simulink model "PV_MEV"  (R2025a)
settings: Solver=VariableStepAuto  StartTime=0.0  StopTime=10.0  RelTol=1e-3
InitFcn:
  | init_paras
values from neighbouring files (symbols this model uses):
  C_PFC = 2600e-6    (= 0.0026)    [init_paras.m]
  chg_ctrl_par = [Icc Vcv V_hys T_hys Kp_v_chg Ki_v_chg Kp_i_chg Ki_i_chg Ts_chg D_max_chg t_chg_on k_chg]    [init_paras.m]
  chg_ev = [0 Icc]    [init_paras.m]
  chg_par = [L_chg Voc Rint Ts_chg I_SIGN t_chg_on]    [init_paras.m]
  D = struct('X', {}, 'ti', {}, 'ia', {}, 'tc', {}, 'irms', {}, 'thd', {}, 'trip', {}, 'ttrip', {})    [make_waveform_figs.m]    (also in run_benchmark.m = get_sig('D'))
  det_ema_alpha = 0.1    [init_paras.m]
  det_force = 0    [init_paras.m]
  det_hyst = 0.6    [init_paras.m]
  det_persist = 2    [init_paras.m]
  det_src = 0    [init_paras.m]
  det_t_arm = 0.58    [init_paras.m]
  det_thr = [0.5 0.5 0.5 0.5 0.5]    [init_paras.m]
  det_variant_onehot = double(det_vlist == VARIANT_NAME)    [init_paras.m]
  ENABLE_HIL = 0    [init_paras.m]
  ENABLE_HIL_DET = 0    [init_paras.m]
  ENABLE_HIL_EST = 0    [init_paras.m]
  estimation_src = cfg_row.estimation_src    [init_paras.m]
  Fnom = 50    [init_paras.m]
  Fr_I = Fnom*2    (= 100)    [init_paras.m]
  grid_df = 0    [init_paras.m]
  grid_h5 = 0    [init_paras.m]
  grid_h7 = 0    [init_paras.m]
  grid_var_t0 = 0.7    [init_paras.m]
  hgq_fusion_alpha = [0.6704476522845647 0.7221651725151749 0.6446423751787858 0.41926421682656173]    [init_paras.m]
  hgq_min_ratio = single(0)    [init_paras.m]
  inj_channel = INJ.channel    [init_paras.m]
  inj_dwell = INJ.dwell    [init_paras.m]
  inj_shape = INJ.shape    [init_paras.m]
  inj_t_on = INJ.t_on    [init_paras.m]
  Ki_V = 80    [init_paras.m]
  Kp_I = 0.06    [init_paras.m]
  Kp_V = 0.25    [init_paras.m]
  Kr_I = 2.5    [init_paras.m]
  L_PFC = 600e-6    (= 0.0006)    [init_paras.m]
  Limit_V = 100    [init_paras.m]
  mit_t_ramp = 0.06    [init_paras.m]
  mitigation_mask = 0    [init_paras.m]
  mm_10cycle_points = mm_points_per_cycle * 10    (= 800)    [init_paras.m]
  mm_fund_freq = 50    [init_paras.m]
  mm_points_per_cycle = 80    [init_paras.m]
  R_bleed = 100e3    (= 100000)    [init_paras.m]
  R_pre = Ro*2    (= 44.44)    [init_paras.m]
  res_par = double(RES.par(:)'); end    [init_paras.m]
  RL_PFC = 20e-3    (= 0.02)    [init_paras.m]
  Ro = 22.22    [init_paras.m]
  t_pre_off = 0.30    (= 0.3)    [init_paras.m]
  Ts_chg = 10e-6    (= 1e-05)    [init_paras.m]
  Ts_Control = 1/Fc    [init_paras.m]
  Ts_Power = 50e-9    (= 5e-08)    [init_paras.m]    (also in run_benchmark.m = evalin('base','Ts_Power'))
  use_d_predict = cfg_row.use_d_predict    [init_paras.m]
  use_detector = 0    [init_paras.m]
  use_harmonic = cfg_row.use_harmonic    [init_paras.m]
  use_p_predict = cfg_row.use_p_predict    [init_paras.m]
  Vnom_ac = 240    [init_paras.m]
  vref_ev = [0 0]    [init_paras.m]
undefined symbols (not defined in the file or in its folder): D1, Delta, DiscIntNeverNeededParam
libraries: spsSeriesRLCBranchLib x17, spsMeanLib x16, MyLibrary x12, spsCurrentMeasurementLib x9, spsFourierLib x8, spsTHDLib x8, spsVoltageMeasurementLib x8, spsDiodeLib x7, simulink x7, pycoexlib x5, instrumentlib x4, spsPWMGeneratorDCDCLib x4
(part 7 of 7)

== matlab function PV_MEV/EV System/PFC Control/D_predict ==
  data: i_L input; D output; i_ref input; V_in input; Ts input; L_in input; V_o input; theta_pll input; amp_est input; phase_est input; use_harmonic input
function D  = fcn(i_L, i_ref, V_in, Ts, L_in, V_o, theta_pll, amp_est, phase_est, use_harmonic)

    persistent theta_prev;
    if isempty(theta_prev)
        theta_prev = theta_pll;
    end

    % hyper parameters
    track_gain = 0.35;
    damp_gain = 0.015;

    % Optional
    lead_steps = 1.0;


    % Initialisation 
    L = max(L_in, 1e-9);
    Ts_eff = max(Ts, 1e-9);
    Vo = max(abs(V_o), 1.0);
    ui_L = max(abs(i_L), 1e-6);

    if V_in > 0
        line_sign = 1.0;
    else
        line_sign = -1.0;
    end

    % Keep the sign of i_ref: a negative reference from the voltage loop must reduce
    % the current (D -> 0, same as the PR controller), not demand |i_ref|.
    i_ref_signed = line_sign * i_ref;

    plant_gain = line_sign * L / (Vo * Ts_eff);
    D_ff = 1.0 - abs(V_in) / Vo;

    if use_harmonic

        dtheta = atan2(sin(theta_pll - theta_prev), cos(theta_pll - theta_prev));
        theta_prev = theta_pll;

        omega_inst = dtheta / Ts_eff;

        theta_ctrl = theta_pll + omega_inst * Ts_eff * lead_steps;

        A3 = abs(amp_est(2));
        A5 = abs(amp_est(3));
        A7 = abs(amp_est(4));

        phi3 = phase_est(1);
        phi5 = phase_est(2);
        phi7 = phase_est(3);

        phase_sign = 1.0;

        ih3 = A3 * sin(3.0 * theta_ctrl + phase_sign * phi3);
        ih5 = A5 * sin(5.0 * theta_ctrl + phase_sign * phi5);
        ih7 = A7 * sin(7.0 * theta_ctrl + phase_sign * phi7);

        k3 = 1.00;
        k5 = 1.08;
        k7 = 1.00;

        ih_357 = k3 * ih3 + k5 * ih5 + k7 * ih7;

        i_ref_signed = i_ref_signed - ih_357;
    end

    i_err = i_ref_signed - i_L;

    D_corr = plant_gain * track_gain * i_err;
    D_damp = -line_sign * damp_gain * (i_L - i_ref_signed) / ui_L;

    D = D_ff + D_corr + D_damp;
end

== matlab function PV_MEV/EV System2/PFC Control/fft estimation 1 cycle2/FFT_estimation_1 ==
  data: u input; amp output; phase output; fs input; f0 input
function [amp, phase] = FFT_estimation_1(u, fs, f0)
%#codegen

x = double(u(:));
N = length(x);

h = zeros(4, 1);
h(1) = 1;
h(2) = 3;
h(3) = 5;
h(4) = 7;

X = fft(x);

amp = zeros(4, 1);
phase_abs_sin = zeros(4, 1);
phase = zeros(3, 1);

tol = 1e-12;

for i = 1:4
    harmonicOrder = h(i);

    bin = round(harmonicOrder * f0 * double(N) / fs);

    if bin <= 0 || bin > floor(double(N) / 2)
        amp(i) = 0;
        phase_abs_sin(i) = 0;
    else
        idx = int32(bin + 1);
        C = X(idx);

        if mod(N, 2) == 0 && bin == N / 2
            amp(i) = abs(C) / double(N);
        else
            amp(i) = 2 * abs(C) / double(N);
        end

        if amp(i) < tol
            phase_abs_sin(i) = 0;
        else
            ph_raw = angle(C);

            ph_sin = ph_raw + pi/2;

            phase_abs_sin(i) = atan2(sin(ph_sin), cos(ph_sin));
        end
    end
end

if amp(1) < tol
    phase(1) = 0;
    phase(2) = 0;
    phase(3) = 0;
else
    phase(1) = atan2( ...
        sin(phase_abs_sin(2) - 3 * phase_abs_sin(1)), ...
        cos(phase_abs_sin(2) - 3 * phase_abs_sin(1)) ...
    );

    phase(2) = atan2( ...
        sin(phase_abs_sin(3) - 5 * phase_abs_sin(1)), ...
        cos(phase_abs_sin(3) - 5 * phase_abs_sin(1)) ...
    );

    phase(3) = atan2( ...
        sin(phase_abs_sin(4) - 7 * phase_abs_sin(1)), ...
        cos(phase_abs_sin(4) - 7 * phase_abs_sin(1)) ...
    );
end

end

== matlab function PV_MEV/EV System2/PFC Control/fft estimation 10 cycle2/FFT_estimation ==
  data: u input; amp output; phase output; fs input; f0 input
function [amp, phase] = FFT_estimation(u, fs, f0)
%#codegen

x = double(u(:));
N = length(x);

h = zeros(4, 1);
h(1) = 1;
h(2) = 3;
h(3) = 5;
h(4) = 7;

X = fft(x);

amp = zeros(4, 1);
phase_abs_sin = zeros(4, 1);
phase = zeros(3, 1);

tol = 1e-12;

for i = 1:4
    harmonicOrder = h(i);

    bin = round(harmonicOrder * f0 * double(N) / fs);

    if bin <= 0 || bin > floor(double(N) / 2)
        amp(i) = 0;
        phase_abs_sin(i) = 0;
    else
        idx = int32(bin + 1);
        C = X(idx);

        if mod(N, 2) == 0 && bin == N / 2
            amp(i) = abs(C) / double(N);
        else
            amp(i) = 2 * abs(C) / double(N);
        end

        if amp(i) < tol
            phase_abs_sin(i) = 0;
        else
            ph_raw = angle(C);

            ph_sin = ph_raw + pi/2;

            phase_abs_sin(i) = atan2(sin(ph_sin), cos(ph_sin));
        end
    end
end

if amp(1) < tol
    phase(1) = 0;
    phase(2) = 0;
    phase(3) = 0;
else
    phase(1) = atan2( ...
        sin(phase_abs_sin(2) - 3 * phase_abs_sin(1)), ...
        cos(phase_abs_sin(2) - 3 * phase_abs_sin(1)) ...
    );

    phase(2) = atan2( ...
        sin(phase_abs_sin(3) - 5 * phase_abs_sin(1)), ...
        cos(phase_abs_sin(3) - 5 * phase_abs_sin(1)) ...
    );

    phase(3) = atan2( ...
        sin(phase_abs_sin(4) - 7 * phase_abs_sin(1)), ...
        cos(phase_abs_sin(4) - 7 * phase_abs_sin(1)) ...
    );
end

end

== matlab function PV_MEV/EV System/PFC Control/HGQ FFT-DL Hybrid ==
  data: fft_amplitude input size=[4 1]; amplitude_out output size=[4 1]; fft_phase input size=[3 1]; dl_amplitude input size=[4 1]; dl_phase input size=[3 1]; alpha input size=[4 1]; minimum_ratio input size=1; phase_out output size=[3 1]; dl_accepted output size=1
function [amplitude_out, phase_out, dl_accepted] = harmonic_hybrid_fusion_block(fft_amplitude, fft_phase, dl_amplitude, dl_phase, alpha, minimum_ratio)
%#codegen
% Fuse FFT (1-cycle) and HGQ2 harmonic estimates in Cartesian coordinates with a
% per-order weight alpha; falls back to FFT when the DL output fails the watchdog.
amplitude_out = zeros(4, 1, 'single');
phase_out = zeros(3, 1, 'single');
dl_accepted = false;
fft_amp = zeros(4, 1, 'single'); dl_amp = zeros(4, 1, 'single'); weight = zeros(4, 1, 'single');
fft_phi = zeros(3, 1, 'single'); dl_phi = zeros(3, 1, 'single');
for index = 1:4
    fft_amp(index) = single(fft_amplitude(index)); dl_amp(index) = single(dl_amplitude(index));
    weight(index) = min(max(single(alpha(index)), single(0)), single(1));
end
for index = 1:3
    fft_phi(index) = single(fft_phase(index)); dl_phi(index) = single(dl_phase(index));
end
ratio = max(single(minimum_ratio), single(0));
valid = true;
for index = 1:4
    valid = valid && isfinite(dl_amp(index)) && dl_amp(index) >= single(0);
end
for index = 1:3
    valid = valid && isfinite(dl_phi(index));
end
valid = valid && dl_amp(1) > single(1e-5);
valid = valid && max(dl_amp(2:4)) <= single(4) * max(dl_amp(1), single(1e-5));
if ~valid
    amplitude_out = fft_amp; phase_out = fft_phi;
    return
end
dl_accepted = true;
amplitude_out(1) = (single(1) - weight(1)) * fft_amp(1) + weight(1) * dl_amp(1);
for index = 1:3
    harmonic = index + 1;
    real_part = (single(1) - weight(harmonic)) * fft_amp(harmonic) * cos(fft_phi(index)) + weight(harmonic) * dl_amp(harmonic) * cos(dl_phi(index));
    imag_part = (single(1) - weight(harmonic)) * fft_amp(harmonic) * sin(fft_phi(index)) + weight(harmonic) * dl_amp(harmonic) * sin(dl_phi(index));
    amplitude_out(harmonic) = hypot(real_part, imag_part);
    phase_out(index) = atan2(imag_part, real_part);
    if amplitude_out(harmonic) < ratio * max(amplitude_out(1), single(1e-5))
        amplitude_out(harmonic) = single(0); phase_out(index) = fft_phi(index);
    end
end
end

== matlab function PV_MEV/EV System/PFC Control/EMI Detector/emi_features ==
  data: X input size=[200 12]; f output size=[1 48]
function f = emi_features(X)
%#codegen
persistent prev
if isempty(prev), prev = zeros(1, 36); end
n = size(X, 1);
vdc = X(:,1); vac = X(:,2); iac = X(:,3); iref = X(:,4); th = X(:,5); d = X(:,6); vr = X(:,7);
vbat = X(:,8); ibat = X(:,9); ddc = X(:,10); st = X(:,11); irb = X(:,12);
k = (0:n-1)';
w1 = 2*pi/n; c1 = cos(w1*k); s1 = sin(w1*k); c2 = cos(2*w1*k); s2 = sin(2*w1*k); c3 = cos(3*w1*k); s3 = sin(3*w1*k);
vac_amp = 2/n*hypot(vac'*c1, vac'*s1); vac_mean = mean(vac);
h1 = 2/n*hypot(iac'*c1, iac'*s1); h2 = 2/n*hypot(iac'*c2, iac'*s2); h3 = 2/n*hypot(iac'*c3, iac'*s3);
iac_mean = mean(iac); iac_rms = sqrt(mean(iac.^2)); pos = max(iac); neg = min(iac);
ref = iref .* abs(sin(th)) .* sign(sin(th));
if std(ref) > 1e-6 && std(iac) > 1e-6, cc = sum((iac-mean(iac)).*(ref-mean(ref))) / (n*std(iac,1)*std(ref,1)); else, cc = 0; end
ref_err = sqrt(mean((abs(iac) - abs(ref)).^2)) / max(iac_rms, 1e-3);
ph_i = atan2(-(iac'*s1), iac'*c1); ph_v = atan2(-(vac'*s1), vac'*c1); dphi = angle(exp(1i*(ph_i - ph_v)));
vdc_mean = mean(vdc); vdc_rip = max(vdc) - min(vdc); vdc_err = vdc_mean - mean(vr);
d_ff = 1 - abs(vac) ./ max(vdc, 50);
p_ac = mean(vac.*iac); p_chg = mean(vbat.*ibat); p_ratio = p_chg / max(p_ac, 50);
vbm = mean(vbat); ddm = mean(ddc);
row = [vac_mean, vac_amp, vac_mean/max(vac_amp,1), iac_mean, iac_rms, pos, neg, pos+neg, h2/max(h1,1e-3), h3/max(h1,1e-3), h1, ...
       cc, ref_err, iac_mean/max(h1,1e-3), dphi, vdc_mean, vdc_rip, vdc_err, mean(iref), min(iref), max(iref), mean(iref < 0), mean(d), mean(d) - mean(d_ff), ...
       vbm, mean(ibat), ddm, mean(st), mean(irb), max(vbat)-min(vbat), max(ibat)-min(ibat), p_ac, p_chg, p_ratio, ...
       ddm*vdc_mean/max(vbm,50) - 1, vbm - ddm*vdc_mean];
if all(prev == 0)
    dl = zeros(1, 7);
else
    dl = [row(16)-prev(16), row(19)-prev(19), row(5)-prev(5), row(4)-prev(4), row(25)-prev(25), row(26)-prev(26), row(34)-prev(34)];
end
prev = row;
% v3 extras (features.FEATURE_NAMES_V3_EXTRA): bus 50 Hz ripple, its ratio to the 100 Hz ripple, its phase vs Vac, duty half-cycle asymmetry, pad
vh1 = 2/n*hypot(vdc'*c1, vdc'*s1); vh2 = 2/n*hypot(vdc'*c2, vdc'*s2);
vph = angle(exp(1i*(atan2(-(vdc'*s1), vdc'*c1) - ph_v)));
sp = sin(th) > 0; sn = sin(th) < 0; dp = 0; dn = 0; if any(sp), dp = mean(d(sp)); end; if any(sn), dn = mean(d(sn)); end
f = [row, dl, vh1, vh1/max(vh2, 0.1), vph, dp - dn, 0];

== matlab function PV_MEV/EV System/PFC Control/EMI Detector/emi_augment ==
  data: f input size=[1 48]; x output size=[1 48]; st input size=[1 49]; onehot input size=[1 6]; alpha input size=1; stn output size=[1 49]
function [x, stn] = emi_augment(f, st, onehot, alpha)
%#codegen
% st = [ema(1:48), n_cycles_seen]
ema = st(1:48); cnt = st(49);
warm = 3;
if cnt < warm
    ema = (ema*cnt + f) / (cnt + 1);      % running mean of the warm-up cycles
    dev = zeros(1, 48);
else
    dev = f - ema;
    ema = (1 - alpha)*ema + alpha*f;
end
stn = [ema, cnt + 1];
x = f;   % 48 base features only (baseline-relative block and one-hot did not help); dev / onehot kept for later

== matlab function PV_MEV/EV System/PFC Control/EMI Detector/emi_decide ==
  data: raw input size=[1 20]; chan output size=[1 5]; thr input size=[1 5]; persist input size=1; cnt input size=[1 5]; hyst input size=1; flag input size=[1 5]; cls output size=1; conf output size=1; amp output size=[1 5]; cntn output size=[1 5]; flagn output size=[1 5]
function [chan, cls, conf, amp, cntn, flagn] = emi_decide(raw, thr, persist, cnt, hyst, flag)
%#codegen
% raw = [5 channel logits, 10 class logits (unused, zeros), 5 signed normalized amplitudes]
% set a channel after `persist` consecutive cycles >= thr, clear it when p < hyst*thr (hysteresis)
pc = 1 ./ (1 + exp(-double(raw(1:5))));
hit = double(pc >= thr); low = double(pc < hyst .* thr);
cntn = (cnt + 1) .* hit;                 % consecutive cycles above threshold
flagn = flag .* (1 - low) + (1 - flag) .* double(cntn >= persist);
chan = flagn;
z = double(raw(6:15)); z = z - max(z); p = exp(z) / sum(exp(z));
[conf, i] = max(p); cls = i - 1;         % 0 none .. 9 multi (features.CLASSES order)
amp = double(raw(16:20)) .* chan;        % per-channel amplitude (Vdc/100 V, Vac/40 V, Iac/20 A, Vbat/25 V, Ibat/8 A), 0 while not flagged

== matlab function PV_MEV/EV System/PFC Control/Mitigation ==
  data: flags input size=[1 5]; Vdc_fb output size=1; amps input size=[1 5]; Vdc input size=1; Vac input size=1; th input size=1; iL input size=1; Iref input size=1; chg input size=[1 9]; mask input size=1; use_det input size=1; force input size=1; Ts input size=1; t_ramp input size=1; Iref_out output size=1; Vin_out output size=1; iL_out output size=1; hold output size=1; g_alpha output size=1; dbg output size=[1 7]; tnow input size=1; t_arm input size=1; inj_ch input size=[1 3]; inj_sh input size=[1 3]; inj_t0 input size=1; inj_dw input size=1; Ilim0 input double size=1; Ilim output double size=1; Vo_ctl output double size=1
function [Vdc_fb, Iref_out, Vin_out, iL_out, hold, g_alpha, dbg, Ilim, Vo_ctl] = mitigation(flags, amps, Vdc, Vac, th, iL, Iref, chg, mask, use_det, force, Ts, t_ramp, tnow, t_arm, inj_ch, inj_sh, inj_t0, inj_dw, Ilim0)
%#codegen
% Detection-conditioned signal corrections for MPCC_R (build_mitigation.m, build_supp.m).  Runs at Ts_Control.
% flags/amps: detector channel flags and signed normalized amplitudes (Vdc Vac Iac Vbat Ibat)
% chg = [Vbat_real Ibat_real Vbat_int Ibat_int D_dcdc state Iref_bat P_charge Idc]
% force = 1: every flag on (MPCC_R_ON); force = 2: oracle flags from the injection definition (MPCC_R_OR)
% M9 (512): slew-limited introduction / removal of the Vdc correction (bumpless), MPCC_R_B
% M11 (2048): protection-consistent voltage-loop limit Ilim = 55 A (OC 65 A less ripple and an uncorrected DC offset) while any correction is active
% M13 (8192): entry-only slew (1000 V/s) of the bus correction during the first 0.1 s after the Vdc flag rises (M9 acts on the fallback path only)
persistent g dVf Iref_prev pkp pkn Vamp th_prev init eb t_rise
if isempty(init), g = zeros(1, 5); dVf = 0; Iref_prev = 0; pkp = 0; pkn = 0; Vamp = 0; th_prev = 0; eb = 0; t_rise = -1; init = 1; end
M = @(k) bitand(uint32(mask), uint32(2^k)) > 0;
f = flags .* (use_det > 0);
if force == 1, f = ones(1, 5); end
if force > 1
    f = zeros(1, 5); dly = 0.02 * round((force - 2) * 10);   % force = 2.d: oracle flags delayed by d grid cycles (fixed-delay oracle)
    if tnow >= inj_t0 + dly && tnow < inj_t0 + inj_dw + dly
        for i = 1:3, c = inj_ch(i); if c >= 1 && c <= 5 && inj_sh(i) ~= 7, f(c) = 1; end, end
    end
end
if tnow < t_arm, f = zeros(1, 5); end          % detector armed only after start-up (det_t_arm)
if f(1) > 0.5, f(4) = 0; f(5) = 0; end         % priority: a Vdc-chain flag explains the charger-side symptoms (Vbat / Ibat flags are consequences)
% --- channel gains: Vdc immediate (a measurement correction must track the bias, not ramp), the rest ramp out over t_ramp (M7)
g1_prev = g(1);
for c = 1:5
    if f(c) > 0.5, g(c) = 1;
    elseif M(7) && c ~= 1, g(c) = max(0, g(c) - Ts / max(t_ramp, Ts));
    else, g(c) = 0; end
end
if g(1) > 0 && g1_prev == 0, t_rise = tnow; end   % rising edge of the bus correction (M13 entry window)
% --- Vdc chain: bias estimate dV = Vdc_int - Vdc_true
Vbat_i = chg(3); Ibat_i = chg(4); Ddc = chg(5);
dV_det = amps(1) * 100;
phys_ok = (Ddc > 0.3) && (Ddc < 0.98) && (Ibat_i > 1);
if phys_ok
    dV = Vdc - Vbat_i / Ddc;                    % charger duty tells the true bus: Vbat = D_dcdc * Vdc_true
else
    dV = dV_det;
end
dV = min(max(dV, -120), 120);
% --- M10 (1024): baseline-referenced estimate.  The residual seen while no bus flag is up is a model-mismatch offset
% (charger losses, parameter error), not a bias: track it slowly (0.2 s) while it moves by less than 5 V, freeze it
% while a flag is up or the residual jumps (an attack), and remove it from the estimate.
if M(10)
    if tnow < t_arm && phys_ok, eb = eb + (Ts / 0.1) * (dV - eb);                                   % calibration before arming
    elseif g(1) == 0 && phys_ok && abs(dV - eb) < 5, eb = eb + (Ts / 0.2) * (dV - eb); end        % slow tracking, jumps excluded
    if phys_ok, dV = min(max(dV - eb, -120), 120); end
end
Vdc_fb = Vdc;
if M(9) && ~phys_ok
    % bumpless: only the amplitude-head fallback is slew-limited (500 V/s); the physics estimate tracks the true bias and
    % vanishes with it, a rate limit there only delays the correction (E-DC-01b: 50 ms of stale correction -> OV)
    tgt = 0; if g(1) > 0, tgt = dV; end
    lim = 500 * Ts; stp = tgt - dVf; stp = min(max(stp, -lim), lim); dVf = dVf + stp;
    if M(0), Vdc_fb = Vdc - dVf; end
else
    if g(1) > 0
        if M(13) && tnow < t_rise + 0.1
            lim = 1000 * Ts; stp = min(max(dV - dVf, -lim), lim); dVf = dVf + stp;   % M13: the correction enters at 1000 V/s, leaves at once
        else, dVf = dVf + (Ts / 0.005) * (dV - dVf); end
    else, dVf = 0; end
    if M(0), Vdc_fb = Vdc - g(1) * dVf; end
end
% --- M11: while a correction is active the voltage loop may not command a current the protection would trip on
Ilim = Ilim0;
if M(11) && (g(1) > 0 || g(4) > 0), Ilim = 55; end   % only the power-moving corrections M0 / M5 (an Ibat / Iac / Vac flag alone leaves the limit at Limit_V)
% --- M14 (16384): the corrected bus sample also feeds the current predictor (its plant model uses V_o); without it a bus bias
% makes the inner loop deliver a current that differs from the reference and the outer loop must over-command (E-DC-02b)
Vo_ctl = Vdc;
if M(14), Vo_ctl = Vdc_fb; end
% --- Iref amplitude limits (M0 floor, M1 slew) live in the separate block 'Mitigation Iref' (algebraic loop)
Iref_out = 0 * Iref + Iref_prev * 0;
% --- Vac chain: PLL-reconstructed feed-forward voltage (peak-to-peak / 2 of the previous cycle)
if th < th_prev - 3                          % wrap: new cycle
    Vamp = 0.5 * (pkp - pkn); pkp = 0; pkn = 0;
end
th_prev = th; pkp = max(pkp, Vac); pkn = min(pkn, Vac);
Vin_out = Vac;
if M(2) && g(2) > 0 && Vamp > 50, Vin_out = Vac + g(2) * (Vamp * sin(th) - Vac); end
% --- Iac chain: DC compensation of the predictor current, estimator hold
iL_out = iL;
if M(3), iL_out = iL - g(3) * amps(3) * 20; end
hold = 0;
if M(4) && g(3) > 0, hold = 1; end
% --- fusion weight towards the HGQ2 estimate while Vac is flagged
g_alpha = 0;
if M(8), g_alpha = g(2); end
dbg = [g(1), dVf, double(phys_ok), Vamp, g(3), eb, Ilim];

== matlab function PV_MEV/EV System/Charger Stage/batt ==
  data: Ibat input double size=1; Vbat output double size=1; pp input double size=[1 6]; P output double size=1
function [Vbat, P] = batt(Ibat, pp)
% Battery terminal voltage and charging power from the current state.
Vbat = pp(2) + pp(3)*Ibat;
P = Vbat*Ibat;

== matlab function PV_MEV/EV System/Charger Stage/ctrl ==
  data: Vbat_m input double size=1; D output double size=1; Ibat_m input double size=1; Vdc input double size=1; t input double size=1; x input double size=[1 5]; pc input double size=[1 13]; ev input double size=[1 2]; Iref output double size=1; xn output double size=[1 5]; state output double size=1
function [D, Iref, xn, state] = ctrl(Vbat_m, Ibat_m, Vdc, t, x, pc, ev)
% CC/CV charge controller.  x = [state tmr xv xi]  (0 CC, 1 CV)
% pc = [Icc Vcv Vhys Thys Kp_v Ki_v Kp_i Ki_i Ts Dmax t_on k_ramp k_soft]; k_soft > 0 (M12): rising slew limit on Iref at every re-engagement
% ev = [t_step Icc_new]: benign charging-current reference step (t_step <= 0: none)
Icc=pc(1); Vcv=pc(2); Vhys=pc(3); Thys=pc(4); Kpv=pc(5); Kiv=pc(6);
Kpi=pc(7); Kii=pc(8); Ts=pc(9); Dmax=pc(10); t_on=pc(11); kr=pc(12); kso=0; if numel(pc) >= 13, kso=pc(13); end
if ev(1) > 0 && t >= ev(1), Icc = ev(2); end
st = x(1); tmr = x(2); xv = x(3); xi = x(4); Iprev = x(5);
Iramp = min(Icc, max(0, (t - t_on)*kr));
% --- state machine
if st == 0
    if Vbat_m >= Vcv, st = 1; tmr = 0; end
else
    if Vbat_m <= Vcv - Vhys, tmr = tmr + Ts; else, tmr = 0; end
    if tmr >= Thys, st = 0; tmr = 0; end
end
% --- outer voltage loop (CV only), preloaded to Iramp in CC
if st == 1
    ev = Vcv - Vbat_m;
    xv = xv + Kiv*ev*Ts;
    Iref = Kpv*ev + xv;
    if Iref > Iramp, Iref = Iramp; xv = min(xv, Iramp); end
    if Iref < 0,     Iref = 0;     xv = max(xv, 0); end
else
    Iref = Iramp; xv = Iramp;
end
if kso > 0 && t >= t_on && Iref > Iprev + kso*Ts, Iref = Iprev + kso*Ts; xv = min(xv, Iref); end   % M12: soft re-engagement
% --- inner current loop with duty feed-forward
ei = Iref - Ibat_m;
xi = xi + Kii*ei*Ts;
Dff = Vbat_m / max(Vdc, 50);
D = Dff + Kpi*ei + xi;
if D > Dmax, D = Dmax; xi = xi - Kii*ei*Ts; end
if D < 0,    D = 0;    xi = xi - Kii*ei*Ts; end
if t < t_on, D = 0; xi = 0; end
xn = [st tmr xv xi Iref];
state = st;

== matlab function PV_MEV/EV System/Charger Stage/plant ==
  data: D input double size=1; Ibat_next output double size=1; Ibat input double size=1; Vdc input double size=1; pp input double size=[1 6]; t input double size=1; Isrc output double size=1; chg_eff parameter double
function [Ibat_next, Isrc] = plant(D, Ibat, Vdc, pp, t, chg_eff)
% Averaged buck.  pp = [L_chg Voc Rint Ts_chg I_SIGN t_chg_on]
% Ibat is the inductor/battery current state (>= 0, diode conduction).
L = pp(1); Voc = pp(2); Rint = pp(3); Ts = pp(4); sgn = pp(5);
Vbat = Voc + Rint*Ibat;
Idc = D*Ibat;                      % lossless averaged input current
Isrc = sgn*Idc;
if t < pp(6)
    Ibat_next = 0;
else
    Ibat_next = Ibat + Ts/L*(chg_eff*D*Vdc - Vbat);   % chg_eff: conversion loss (model-mismatch test)
    if Ibat_next < 0, Ibat_next = 0; end
end

== matlab function PV_MEV/EV System/Charger Stage/chg_corr ==
  data: Vbat_m input size=1; Vbat_c output size=1; Ibat_m input size=1; flags input size=[1 5]; amps input size=[1 5]; mask input size=1; use_det input size=1; force input size=1; Ts input size=1; t_ramp input size=1; Ibat_c output size=1; tnow input size=1; t_arm input size=1; Vdc input size=1; D_prev input size=1; inj_ch input size=[1 3]; inj_sh input size=[1 3]; inj_t0 input size=1; inj_dw input size=1
function [Vbat_c, Ibat_c] = chg_corr(Vbat_m, Ibat_m, flags, amps, mask, use_det, force, Ts, t_ramp, tnow, t_arm, Vdc, D_prev, inj_ch, inj_sh, inj_t0, inj_dw)
%#codegen
% M5 / M6: remove the detected Vbat / Ibat measurement bias before the CC/CV controller (build_mitigation.m, build_supp.m)
% force = 2: oracle flags from the injection definition; M9 (512): slew-limited (200 V/s) Vbat correction
persistent g dVf init eb
if isempty(init), g = zeros(1, 2); dVf = 0; eb = 0; init = 1; end
fl = flags .* (use_det > 0);
if force == 1, fl = ones(1, 5); end
if force > 1
    fl = zeros(1, 5); dly = 0.02 * round((force - 2) * 10);
    if tnow >= inj_t0 + dly && tnow < inj_t0 + inj_dw + dly
        for i = 1:3, c = inj_ch(i); if c >= 1 && c <= 5 && inj_sh(i) ~= 7, fl(c) = 1; end, end
    end
end
f = fl(4:5);
if tnow < t_arm || fl(1) > 0.5, f = zeros(1, 2); end   % armed after start-up; a Vdc-chain flag overrides the charger-side flags
ramp = bitand(uint32(mask), uint32(128)) > 0;
for c = 1:2
    if f(c) > 0.5, g(c) = 1;
    elseif ramp, g(c) = max(0, g(c) - Ts / max(t_ramp, Ts));
    else, g(c) = 0; end
end
Vbat_c = Vbat_m; Ibat_c = Ibat_m;
phys_ok = (D_prev > 0.3) && (D_prev < 0.98) && (Ibat_m > 1) && (Vdc > 250);
if phys_ok, dV = Vbat_m - D_prev * Vdc; else, dV = amps(4) * 25; end   % buck: Vbat = D * Vdc while regulating; detector amplitude as fallback
dV = min(max(dV, -60), 60);
if bitand(uint32(mask), uint32(1024)) > 0      % M10: baseline-referenced (model-mismatch offset removed), see Mitigation
    if tnow < t_arm && phys_ok, eb = eb + (Ts / 0.1) * (dV - eb);
    elseif g(1) == 0 && phys_ok && abs(dV - eb) < 3, eb = eb + (Ts / 0.2) * (dV - eb); end
    if phys_ok, dV = min(max(dV - eb, -60), 60); end
end
if bitand(uint32(mask), uint32(512)) > 0 && ~phys_ok      % M9: slew-limited amplitude-head fallback only (100 V/s)
    tgt = 0; if g(1) > 0, tgt = dV; end
    lim = 100 * Ts; stp = tgt - dVf; stp = min(max(stp, -lim), lim); dVf = dVf + stp;
    if bitand(uint32(mask), uint32(32)) > 0, Vbat_c = Vbat_m - dVf; end
else
    if g(1) > 0, dVf = dVf + (Ts / 0.002) * (dV - dVf); else, dVf = 0; end
    if bitand(uint32(mask), uint32(32)) > 0, Vbat_c = Vbat_m - g(1) * dVf; end
end
if bitand(uint32(mask), uint32(64)) > 0, Ibat_c = Ibat_m - g(2) * amps(5) * 8; end

== matlab function PV_MEV/EV System/PFC Control/UMPC Function Full bridge1 ==
  data: i_L input; y output; i_ref input; V_in input; Ts input; L_in input; V_o input; g_on output; g_off output
function [y,g_on,g_off]= fcn(i_L, i_ref, V_in, Ts, L_in, V_o)

    L=L_in;

    if V_in >= 0
        i_ref_signed = i_ref;
    else
        i_ref_signed = -i_ref;
    end;

    % -- Positive half Cycle
    if V_in >0
        % --- Candidate 1: Switch ON ---
        g_on  = i_L + (V_in)*Ts/L;
        e_on  = abs(g_on - i_ref_signed);
        
        % --- Candidate 2: Switch OFF ---
        g_off = i_L + (V_in - V_o)*Ts/L;
        e_off = abs(g_off - i_ref_signed);

     % -- Negative half Cycle
    else
        % --- Candidate 1: Switch ON ---
        g_on  = i_L + (V_in)*Ts/L;
        e_on  = abs(g_on - i_ref_signed);

        % --- Candidate 2: Switch OFF ---
        g_off = i_L + (V_in + V_o)*Ts/L;
        e_off = abs(g_off - i_ref_signed);
    end

    % --- MPC Decision: pick action with lower predicted error ---
    if e_on <= e_off
        y = true;
    else
        y = false;
    end

== matlab function PV_MEV/EV System/PFC Control/Mitigation Iref ==
  data: Iref input size=1; Iref_out output size=1; dbg input size=[1 7]; mask input size=1; Ts input size=1
function Iref_out = mitigation_iref(Iref, dbg, mask, Ts)
%#codegen
% M0: no negative reference while the Vdc chain is flagged; M1: slew-rate limit (200 A/s) while flagged.
% g_vdc = dbg(1) is the ramped Vdc-chain gain of the Mitigation block (build_mitigation.m).
persistent Iref_prev init
if isempty(init), Iref_prev = 0; init = 1; end
g1 = dbg(1);
Iref_out = Iref;
if bitand(uint32(mask), uint32(1)) > 0 && g1 > 0, Iref_out = max(Iref_out, 0); end
if bitand(uint32(mask), uint32(2)) > 0 && g1 > 0
    dmax = 200 * Ts;
    Iref_out = min(max(Iref_out, Iref_prev - dmax), Iref_prev + dmax);
end
Iref_prev = Iref_out;

== matlab function PV_MEV/EV System/PFC Control/hil_flagword ==
  data: c input size=[1 5]; w output size=1
function w = flagword(c)
%#codegen
w = single(c(1) + 2*c(2) + 4*c(3) + 8*c(4) + 16*c(5));

== matlab function PV_MEV/EV System/PFC Control/HIL MPCC TCP ==
  data: x input; y output double size=[1 1]
function y = hil_mpcc_tcp(x)
%#codegen
coder.extrinsic('hil_tcp');
xd = double(x);
yd = zeros(1, 1);
yd = hil_tcp(xd, 1, 5010, 5011);
y = cast(yd, 'double');

== matlab function PV_MEV/EV System/PFC Control/EMI Detector/HIL Det TCP ==
  data: x input; y output single size=[1 21]
function y = hil_det_tcp(x)
%#codegen
coder.extrinsic('hil_tcp');
xd = double(x);
yd = zeros(1, 21);
yd = hil_tcp(xd, 21, 5020, 5021);
y = cast(yd, 'single');

== matlab function PV_MEV/EV System/PFC Control/One  Cycle Model Prediction/HIL Est TCP ==
  data: x input; y output single size=[1 8]
function y = hil_est_tcp(x)
%#codegen
coder.extrinsic('hil_tcp');
xd = double(x);
yd = zeros(1, 8);
yd = hil_tcp(xd, 8, 5030, 5031);
y = cast(yd, 'single');

== matlab function PV_MEV/EV System/PFC Control/tick_hold ==
  data: D input; Dout output; hold input
function Dout = tick_hold(D, hold)
%#codegen
% hold the previous duty on ticks the measured PS schedule marked late (review-2 point 6)
persistent Dprev init
if isempty(init), Dprev = 0; init = 1; end
if hold > 0.5, Dout = Dprev; else, Dout = D; end
Dprev = Dout;

== matlab function PV_MEV/EV System/PFC Control/EMI Detector/residual_score ==
  data: feat input single size=[1 48]; raw output single size=[1 20]; par input double size=[1 53]
function raw = residual_score(feat, par)
%#codegen
% joint-residual baseline of detector_eval_unified.py (export_residual.py): |x - med| / mad on six residual features,
% one logistic regression per channel; the same decision block, thresholds (RES.thr) and corrections follow.
f = double(feat(:)'); med = par(7:12); mad = par(13:18); W = reshape(par(19:48), 6, 5); b = par(49:53);
z = zeros(1, 6);
for k = 1:6
    i = min(48, max(1, round(par(k))));   % feature index (1-based); res_par is all zeros when the network is the source
    z(k) = abs(f(i) - med(k)) / max(mad(k), 1e-6);
end
lg = z * W + b;
raw = single([lg, zeros(1, 10), zeros(1, 5)]);

== matlab function PV_MEV/EV System/PFC Control/One  Cycle Model Prediction/MATLAB Function3 ==
  data: y_encoded input; y_post output; window_peak input; ema_alpha input; reset input
function y_post = harmonic_postprocess8_block(y_encoded, window_peak, ema_alpha, reset)
%#codegen
% Decode [c1,s1,c3,s3,c5,s5,c7,s7] to the legacy MPCC vector [A1,A3,A5,A7,delta3,delta5,delta7]
% (same as the packaged FFT_HGQ_BLS model; window_peak is the CycleNorm side channel).
persistent state initialized
if isempty(initialized)
    state = zeros(8, 1, 'single');
    initialized = false;
end
y = zeros(8, 1, 'single');
for index = 1:8
    y(index) = single(y_encoded(index));
end
alpha = min(max(single(ema_alpha), single(0)), single(1));
if ~initialized || reset ~= 0
    state = y;
    initialized = true;
else
    state = alpha * y + (single(1) - alpha) * state;
end
peak = max(abs(single(window_peak)), single(1e-6));
order_scale = single([1.0; 0.25; 0.20; 0.15]);
amplitude = zeros(4, 1, 'single');
phase = zeros(4, 1, 'single');
for harmonic_index = 1:4
    component = 2 * harmonic_index - 1;
    real_part = state(component);
    imag_part = state(component + 1);
    amplitude(harmonic_index) = peak * order_scale(harmonic_index) * hypot(real_part, imag_part);
    phase(harmonic_index) = atan2(imag_part, real_part);
end
orders = single([3; 5; 7]);
y_post = zeros(7, 1, 'single');
y_post(1:4) = amplitude;
for index = 1:3
    relative = phase(index + 1) - orders(index) * phase(1);
    y_post(index + 4) = atan2(sin(relative), cos(relative));
end
end

== matlab function PV_MEV/EV System/PFC Control/Half Cycle Model Prediction/MATLAB Function ==
  data: x input; x_norm output; A output
function [x_norm, A] = CycleNorm(x)
A = max(abs(x));
A = max(A, 1e-6);
x_norm = x / A;

== matlab function PV_MEV/EV System/PFC Control/Half Cycle Model Prediction/MATLAB Function3 ==
  data: y_rel input; y_post output; A_latest input; alpha input; reset input
function y_post = harmonic_postprocess(y_rel, A_latest, alpha, reset)
%#codegen
% 一体化后处理：
% 1) EMA 平滑（在相对输出域）
% 2) A 恢复（幅值乘 A）
% 3) atan2 恢复相位（由 cos/sin -> phase）
%
% 输入:
%   y_rel    : 模型输出(10x1 或 1x10)
%              [amp_h1_rel, amp_h3_rel, amp_h5_rel, amp_h7_rel, ...
%               cos_h3, sin_h3, cos_h5, sin_h5, cos_h7, sin_h7]
%   A_latest : A 恢复系数（可标量或向量；向量时自动取 max(abs(.))）
%   alpha    : EMA 系数 [0,1]，建议 0.10~0.16
%   reset    : 复位信号（true 时重置 EMA 状态）
%
% 输出:
%   y_post(7x1):
%   [amp_h1_abs, amp_h3_abs, amp_h5_abs, amp_h7_abs, phase_h3, phase_h5, phase_h7]

persistent ema_state initialized
if isempty(initialized)
    ema_state = zeros(10,1,'single');
    initialized = false;
end

% -------- 参数/输入整理 --------
y = zeros(10,1,'single');
for i = 1:10
    y(i) = single(y_rel(i));
end

a = single(abs(A_latest));
if numel(a) > 1
    a = max(a(:));
end
if a < single(1e-6)
    a = single(1e-6);
end

a_ema = single(alpha);
if a_ema < single(0)
    a_ema = single(0);
elseif a_ema > single(1)
    a_ema = single(1);
end

do_reset = (reset ~= 0);

% -------- EMA --------
if ~initialized || do_reset
    ema_state = y;
    initialized = true;
else
    ema_state = a_ema * y + (single(1) - a_ema) * ema_state;
end

% -------- A 恢复（幅值）--------
amp = ema_state(1:4) * a;

% -------- 相位恢复（cos/sin -> atan2）--------
% 先单位化，避免 cos/sin 长度漂移导致相位抖动
c3 = ema_state(5); s3 = ema_state(6);
n3 = sqrt(c3*c3 + s3*s3); if n3 < single(1e-6), n3 = single(1e-6); end
c3 = c3 / n3; s3 = s3 / n3;

c5 = ema_state(7); s5 = ema_state(8);
n5 = sqrt(c5*c5 + s5*s5); if n5 < single(1e-6), n5 = single(1e-6); end
c5 = c5 / n5; s5 = s5 / n5;

c7 = ema_state(9); s7 = ema_state(10);
n7 = sqrt(c7*c7 + s7*s7); if n7 < single(1e-6), n7 = single(1e-6); end
c7 = c7 / n7; s7 = s7 / n7;

ph3 = atan2(s3, c3);
ph5 = atan2(s5, c5);
ph7 = atan2(s7, c7);

% -------- 最终输出（仅最终量）--------
y_post = zeros(7,1,'single');
y_post(1:4) = amp;
y_post(5) = ph3;
y_post(6) = ph5;
y_post(7) = ph7;

end

== matlab function PV_MEV/EV System/PFC Control/MCP Function Half bridge1 ==
  data: i_L input; y output; i_ref input; V_in input; Ts input; L_in input; V_o input
function y = fcn(i_L, i_ref, V_in, Ts, L_in, V_o)

    L=2*pi*50*L_in;
    % --- Candidate 1: Switch ON ---
    g_on  = i_L + abs(V_in)*Ts/L;
    e_on  = abs(g_on - i_ref);

    % --- Candidate 2: Switch OFF ---
    g_off = i_L + (abs(V_in)-V_o)*Ts/L;
    e_off = abs(g_off - i_ref);

    % --- MPC Decision: pick action with lower predicted error ---
    if e_on <= e_off
        y = true;
    else
        y = false;
    end
